simulink library "AllocatorsLib"  (R2022b)
settings: Solver=VariableStepAuto  StartTime=0.0  StopTime=10.0  RelTol=1e-3
libraries: ComponentsLib x7
settings Model: Creator=tbritton  LastModifiedBy=macheson
settings SolverCC: AlgebraicLoopSolver=TrustRegion
settings DebuggingCC: UnconnectedInputMsg=warning  UnconnectedOutputMsg=warning  UnconnectedLineMsg=warning  SFMachineParentedDataDiag=warning
settings ModelReferenceCC: EnableRefExpFcnMdlSchedulingChecks=on
settings RTWCC: DLArmComputeVersion=19.05

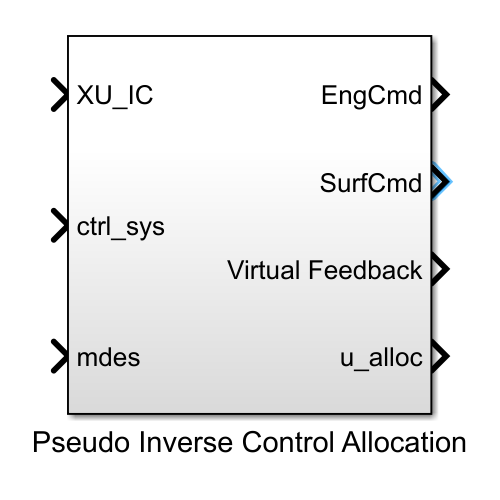
[thumbnail: Simulink's stored preview of the top-level diagram]
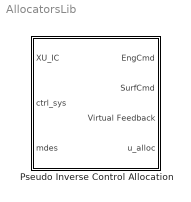
== system AllocatorsLib ==
  Pseudo Inverse Control Allocation : Subsystem

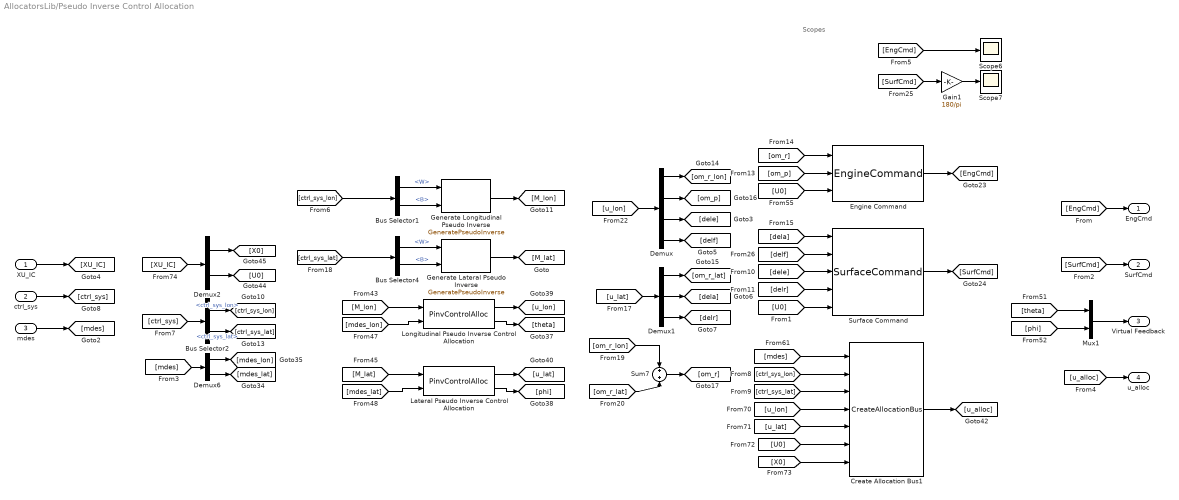
== system AllocatorsLib/Pseudo Inverse Control Allocation ==
  note: Scopes
  XU_IC : Inport
  ctrl_sys : Inport  Port=2
  mdes : Inport  Port=3
  Bus Selector1 : BusSelector  OutputSignals=W,B
  Bus Selector2 : BusSelector  OutputSignals=ctrl_sys_lon,ctrl_sys_lat
  Bus Selector4 : BusSelector  OutputSignals=W,B
  Create Allocation Bus1 : ComponentsLib/CreateAllocationBus  SystemSampleTime=-1  VariantActivationTime=update diagram  Latency=0  AutoFrameSizeCalculation=off
      settings: SourceProductName=GUAM Controller Blockset
  Demux : Demux  Outputs=[8 1 1 1]
  Demux1 : Demux  Outputs=[8 1 1]
  Demux2 : Demux  Outputs=[12 13]
  Demux6 : Demux  Outputs=[3 3]
  Engine Command : ComponentsLib/EngineCommand  SystemSampleTime=-1  VariantActivationTime=update diagram  Latency=0  AutoFrameSizeCalculation=off
      settings: SourceProductName=GUAM Controller Blockset
  Gain1 : Gain  Gain=180/pi
  Generate Lateral Pseudo Inverse : ComponentsLib/GeneratePseudoInverse  SystemSampleTime=-1  VariantActivationTime=update diagram  Latency=0  AutoFrameSizeCalculation=off
      settings: SourceProductName=GUAM Controller Blockset
  Generate Longitudinal Pseudo Inverse : ComponentsLib/GeneratePseudoInverse  SystemSampleTime=-1  VariantActivationTime=update diagram  Latency=0  AutoFrameSizeCalculation=off
      settings: SourceProductName=GUAM Controller Blockset
  Lateral Pseudo Inverse Control Allocation : ComponentsLib/PinvControlAlloc  SystemSampleTime=-1  VariantActivationTime=update diagram  Latency=0  AutoFrameSizeCalculation=off
      settings: SourceProductName=GUAM Controller Blockset
  Longitudinal Pseudo Inverse Control Allocation : ComponentsLib/PinvControlAlloc  SystemSampleTime=-1  VariantActivationTime=update diagram  Latency=0  AutoFrameSizeCalculation=off
      settings: SourceProductName=GUAM Controller Blockset
  Mux1 : Mux  Inputs=2
  Scope6 : Scope
  Scope7 : Scope
  Sum7 : Sum
  Surface Command : ComponentsLib/SurfaceCommand  SystemSampleTime=-1  VariantActivationTime=update diagram  Latency=0  AutoFrameSizeCalculation=off
      settings: SourceProductName=GUAM Controller Blockset
  EngCmd : Outport
  SurfCmd : Outport  Port=2
  Virtual Feedback : Outport  Port=3
  u_alloc : Outport  Port=4
  wires:
  Lateral Pseudo Inverse Control Allocation/2 -> [phi]
  Longitudinal Pseudo Inverse Control Allocation/1 -> [u_lon]
  [theta] -> Mux1/1
  [mdes_lat] -> Lateral Pseudo Inverse Control Allocation/2
  [phi] -> Mux1/2
  [mdes_lon] -> Longitudinal Pseudo Inverse Control Allocation/2
  Lateral Pseudo Inverse Control Allocation/1 -> [u_lat]
  Longitudinal Pseudo Inverse Control Allocation/2 -> [theta]
  Mux1/1 -> Virtual Feedback/1
  [M_lon] -> Longitudinal Pseudo Inverse Control Allocation/1
  [M_lat] -> Lateral Pseudo Inverse Control Allocation/1
  Demux/3 -> [dele]
  Demux/2 -> [om_p]
  [u_lat] -> Demux1/1
  [om_r_lat] -> Sum7/2
  [om_r_lon] -> Sum7/1
  Sum7/1 -> [om_r]
  [u_lon] -> Demux/1
  Demux1/2 -> [dela]
  Demux1/1 -> [om_r_lat]
  Demux/1 -> [om_r_lon]
  Demux/4 -> [delf]
  Demux1/3 -> [delr]
  Engine Command/1 -> [EngCmd]
  Surface Command/1 -> [SurfCmd]
  [U0] -> Engine Command/3
  [dele] -> Surface Command/3
  [delf] -> Surface Command/2
  [delr] -> Surface Command/4
  [om_p] -> Engine Command/2
  [om_r] -> Engine Command/1
  [U0] -> Surface Command/5
  [dela] -> Surface Command/1
  [EngCmd] -> EngCmd/1
  [SurfCmd] -> SurfCmd/1
  Demux2/2 -> [U0]
  [U0] -> Create Allocation Bus1/6
  [u_lon] -> Create Allocation Bus1/4
  Create Allocation Bus1/1 -> [u_alloc]
  [u_lat] -> Create Allocation Bus1/5
  [XU_IC] -> Demux2/1
  [X0] -> Create Allocation Bus1/7
  Demux2/1 -> [X0]
  [mdes] -> Create Allocation Bus1/1
  Demux6/2 -> [mdes_lat]
  Demux6/1 -> [mdes_lon]
  [mdes] -> Demux6/1
  mdes/1 -> [mdes]
  XU_IC/1 -> [XU_IC]
  ctrl_sys/1 -> [ctrl_sys]
  [u_alloc] -> u_alloc/1
  Gain1/1 -> Scope7/1
  [SurfCmd] -> Gain1/1
  [EngCmd] -> Scope6/1
  [ctrl_sys_lat] -> Bus Selector4/1
  Bus Selector1/1 -> Generate Longitudinal Pseudo Inverse/1  "<W>"
  [ctrl_sys_lon] -> Bus Selector1/1
  Generate Longitudinal Pseudo Inverse/1 -> [M_lon]
  Bus Selector4/1 -> Generate Lateral Pseudo Inverse/1  "<W>"
  Generate Lateral Pseudo Inverse/1 -> [M_lat]
  Bus Selector4/2 -> Generate Lateral Pseudo Inverse/2  "<B>"
  Bus Selector1/2 -> Generate Longitudinal Pseudo Inverse/2  "<B>"
  [ctrl_sys] -> Bus Selector2/1
  Bus Selector2/1 -> [ctrl_sys_lon]  "<ctrl_sys_lon>"
  Bus Selector2/2 -> [ctrl_sys_lat]  "<ctrl_sys_lat>"
  [ctrl_sys_lon] -> Create Allocation Bus1/2
  [ctrl_sys_lat] -> Create Allocation Bus1/3
